simulink model "CC"  (R2014b)
settings: Solver=FixedStepAuto  StartTime=0.0  StopTime=10  FixedStep=0.12  RelTol=1e-3  EnableMultiTasking=on
values from neighbouring files (symbols this model uses):
  Adk = Ad-Bd*Koc    [l1.m]
  Bdk = Bd*Rpr    [l1.m]
  Cdk = Cd    [l1.m]
  Koc = place(Ad,Bd,p)    [l1.m]
undefined symbols (not defined in the file or in its folder): A, Ad, B, Bd, C, Cd
settings Model: Creator=Admin  LastModifiedBy=Student
settings OptimizationCC: UseDivisionForNetSlopeComputation=off  SimCompilerOptimization=off
settings DebuggingCC: SolverPrmCheckMsg=none  FcnCallInpInsideContextMsg=error  FrameProcessingCompatibilityMsg=error  SFExecutionAtInitializationDiag=none
settings HardwareCC: ProdBitPerSizeT=32  ProdBitPerPtrDiffT=32
settings RTWCC: RTWCompilerOptimization=off
settings ConfigComp: CovMetricSettings=dw  CovHtmlReporting=on  CovSaveCumulativeToWorkspaceVar=on  CovSaveSingleToWorkspaceVar=on  CovExternalEMLEnable=off  CovSFcnEnable=off

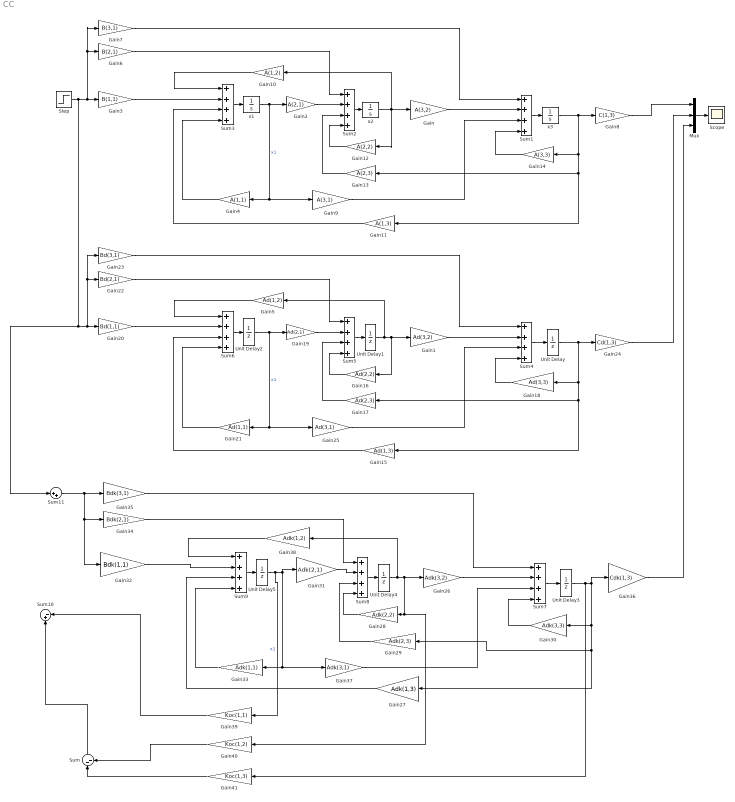
== system CC ==
  Gain : Gain  Gain=A(3,2)
  Gain1 : Gain  Gain=Ad(3,2)
  Gain10 : Gain  Gain=A(1,2)
  Gain11 : Gain  Gain=A(1,3)
  Gain12 : Gain  Gain=A(2,2)
  Gain13 : Gain  Gain=A(2,3)
  Gain14 : Gain  Gain=A(3,3)
  Gain15 : Gain  Gain=Ad(1,3)
  Gain16 : Gain  Gain=Ad(2,2)
  Gain17 : Gain  Gain=Ad(2,3)
  Gain18 : Gain  Gain=Ad(3,3)
  Gain19 : Gain  Gain=Ad(2,1)
  Gain2 : Gain  Gain=A(2,1)
  Gain20 : Gain  Gain=Bd(1,1)
  Gain21 : Gain  Gain=Ad(1,1)
  Gain22 : Gain  Gain=Bd(2,1)
  Gain23 : Gain  Gain=Bd(3,1)
  Gain24 : Gain  Gain=Cd(1,3)
  Gain25 : Gain  Gain=Ad(3,1)
  Gain26 : Gain  Gain=Adk(3,2)
  Gain27 : Gain  Gain=Adk(1,3)
  Gain28 : Gain  Gain=Adk(2,2)
  Gain29 : Gain  Gain=Adk(2,3)
  Gain3 : Gain  Gain=B(1,1)
  Gain30 : Gain  Gain=Adk(3,3)
  Gain31 : Gain  Gain=Adk(2,1)
  Gain32 : Gain  Gain=Bdk(1,1)
  Gain33 : Gain  Gain=Adk(1,1)
  Gain34 : Gain  Gain=Bdk(2,1)
  Gain35 : Gain  Gain=Bdk(3,1)
  Gain36 : Gain  Gain=Cdk(1,3)
  Gain37 : Gain  Gain=Adk(3,1)
  Gain38 : Gain  Gain=Adk(1,2)
  Gain39 : Gain  Gain=Koc(1,1)
  Gain4 : Gain  Gain=A(1,1)
  Gain40 : Gain  Gain=Koc(1,2)
  Gain41 : Gain  Gain=Koc(1,3)
  Gain5 : Gain  Gain=Ad(1,2)
  Gain6 : Gain  Gain=B(2,1)
  Gain7 : Gain  Gain=B(3,1)
  Gain8 : Gain  Gain=C(1,3)
  Gain9 : Gain  Gain=A(3,1)
  Mux : Mux  Inputs=3
  Scope : Scope
  Step : Step  Time=0  SampleTime=0
  Sum : Sum  Inputs=|--
  Sum{1..9} (9 alike) : Sum  Inputs=++++
  Sum10 : Sum  Inputs=|+-
  Sum11 : Sum  Inputs=|++
  Unit Delay{,1..5} (6 alike) : UnitDelay  SampleTime=-1
  x1 : Integrator
  x2 : Integrator
  x3 : Integrator
  wires:
  Sum1/1 -> x3/1
  Sum2/1 -> x2/1
  Sum3/1 -> x1/1
  Gain2/1 -> Sum2/2
  x1/1 -> Gain9/1, Gain4/1, Gain2/1  "x1"
  x2/1 -> Gain12/1, Gain/1, Gain10/1
  Gain/1 -> Sum1/2
  x3/1 -> Gain14/1, Gain11/1, Gain13/1, Gain8/1
  Gain3/1 -> Sum3/2
  Gain6/1 -> Sum2/1
  Gain7/1 -> Sum1/1
  Gain8/1 -> Mux/1
  Gain4/1 -> Sum3/4
  Gain9/1 -> Sum1/3
  Gain10/1 -> Sum3/1
  Gain11/1 -> Sum3/3
  Gain12/1 -> Sum2/4
  Gain13/1 -> Sum2/3
  Gain14/1 -> Sum1/4
  Gain25/1 -> Sum4/3
  Gain17/1 -> Sum5/3
  Gain15/1 -> Sum6/3
  Gain5/1 -> Sum6/1
  Gain23/1 -> Sum4/1
  Gain21/1 -> Sum6/4
  Gain22/1 -> Sum5/1
  Unit Delay/1 -> Gain18/1, Gain15/1, Gain17/1, Gain24/1
  Gain18/1 -> Sum4/4
  Gain16/1 -> Sum5/4
  Gain20/1 -> Sum6/2
  Gain1/1 -> Sum4/2
  Sum4/1 -> Unit Delay/1
  Gain19/1 -> Sum5/2
  Unit Delay2/1 -> Gain25/1, Gain21/1, Gain19/1  "x1"
  Unit Delay1/1 -> Gain5/1, Gain16/1, Gain1/1
  Sum5/1 -> Unit Delay1/1
  Sum6/1 -> Unit Delay2/1
  Gain24/1 -> Mux/2
  Gain37/1 -> Sum7/3
  Gain29/1 -> Sum8/3
  Gain27/1 -> Sum9/3
  Gain38/1 -> Sum9/1
  Gain35/1 -> Sum7/1
  Gain33/1 -> Sum9/4
  Gain34/1 -> Sum8/1
  Unit Delay3/1 -> Gain41/1, Gain30/1, Gain27/1, Gain29/1, Gain36/1
  Gain30/1 -> Sum7/4
  Gain28/1 -> Sum8/4
  Gain32/1 -> Sum9/2
  Gain26/1 -> Sum7/2
  Sum7/1 -> Unit Delay3/1
  Gain31/1 -> Sum8/2
  Unit Delay5/1 -> Gain39/1, Gain37/1, Gain33/1, Gain31/1  "x1"
  Unit Delay4/1 -> Gain38/1, Gain40/1, Gain28/1, Gain26/1
  Sum8/1 -> Unit Delay4/1
  Sum9/1 -> Unit Delay5/1
  Step/1 -> Sum11/1, Gain23/1, Gain22/1, Gain20/1, Gain7/1, Gain6/1, Gain3/1
  Gain36/1 -> Mux/3
  Mux/1 -> Scope/1
  Gain39/1 -> Sum10/2
  Gain41/1 -> Sum/1
  Gain40/1 -> Sum/2
  Sum/1 -> Sum10/1
  Sum11/1 -> Gain32/1, Gain34/1, Gain35/1
